simulink model "linear_model_with_controller"  (R2022b)
settings: Solver=VariableStepAuto  StartTime=0.0  StopTime=80  RelTol=1e-3
values from neighbouring files (symbols this model uses):
  A = [-3.78172659857e-08 0 0 0 2.97308e-08 0 0 0 0 1 5.79554624069e-35 6.21514719717e-19 ... (144 elements, 12x12)]    [A1.mat]    (also in A2.mat = [-3.78172659857e-08 0 0 0 2.97308e-08 0 0 0 0 1 -4.775625166; A3.mat = [-3.78172659857e-08 0 0 0 2.97308e-08 0 0 0 0 1 1.7488204834; A4.mat = [-3.78172659857e-08 0 0 0 2.97308e-08 0 0 0 0 1 -4.775625166)
  B = [-5.75123705385 0 0 0 10.0487888864 0 0 0 0 0 0 0 ... (48 elements, 12x4)]    [B1.mat]    (also in B2.mat = [-5.75123707143 0 0 0 10.0487889171 0 0 0 0 0 0 0 ... (48 el; B3.mat = [-5.75123705387 0 0 0 10.0487888865 0 0 0 0 0 0 0 ... (48 el; B4.mat = [-5.75123707143 0 0 0 10.0487889171 0 0 0 0 0 0 0 ... (48 el)
  Lcont = -inv(Sreg*Breg)*((Sreg*Areg)-(Phi*Sreg))*Tr    [Sliding_surface_design.m]
  S = [Mc eye(mm)]*Tr    [Sliding_surface_design.m]
undefined symbols (not defined in the file or in its folder): C, D
settings Model: Creator=henrr  LastModifiedBy=henrr
settings DataIOCC: SaveOutput=off  SaveTime=off  ReturnWorkspaceOutputs=off

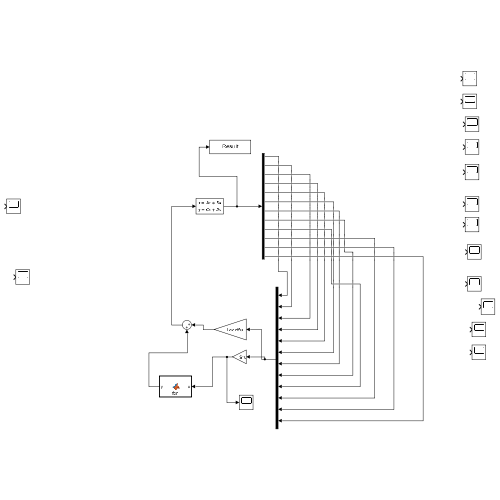
[thumbnail: Simulink's stored preview of the top-level diagram]
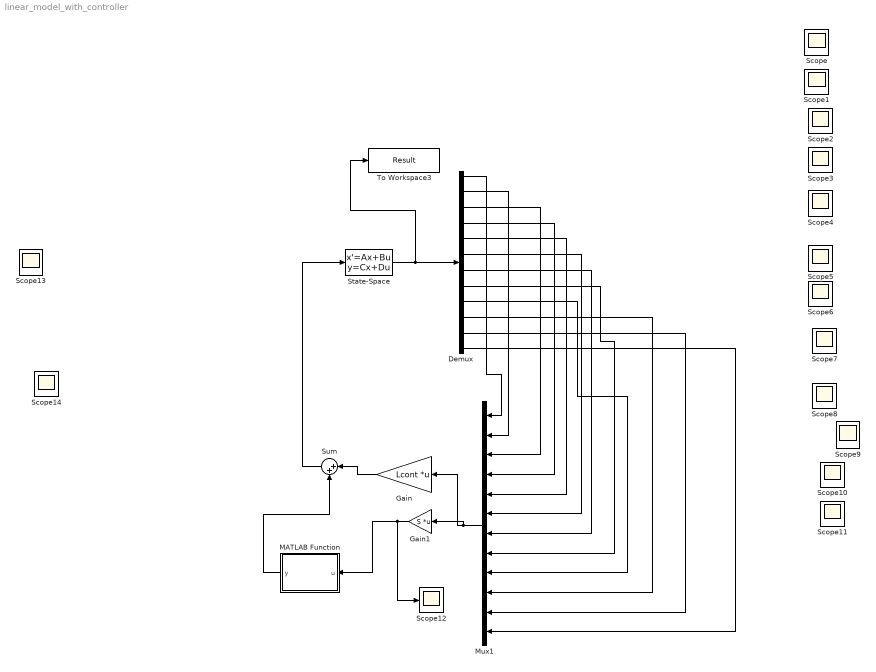
== system linear_model_with_controller ==
  Demux : Demux  Outputs=12
  Gain : Gain  Gain=Lcont  Multiplication=Matrix(K*u)
  Gain1 : Gain  Gain=S  Multiplication=Matrix(K*u)
  MATLAB Function : MATLAB Function  TreatAsAtomicUnit=on
  Mux1 : Mux  Inputs=12
  Scope{,1..14} (15 alike) : Scope
  State-Space : StateSpace  A=A  B=B  C=C  D=D  InitialCondition=[0.1,0,0,0,0,0,0,0,0,0,0,0]'  AllowTunableDMatrix=on
  Sum : Sum  Inputs=|++
  To Workspace3 : ToWorkspace  VariableName=Result  SaveFormat=Timeseries  SampleTime=-1
  wires:
  Demux/9 -> Mux1/9
  Demux/7 -> Mux1/7
  Demux/12 -> Mux1/12
  Demux/8 -> Mux1/8
  Demux/1 -> Mux1/1
  Demux/6 -> Mux1/6
  Demux/2 -> Mux1/2
  Demux/11 -> Mux1/11
  Demux/4 -> Mux1/4
  Demux/10 -> Mux1/10
  Demux/5 -> Mux1/5
  State-Space/1 -> To Workspace3/1, Demux/1
  Gain1/1 -> Scope12/1, MATLAB Function/1(u)
  Sum/1 -> State-Space/1
  Demux/3 -> Mux1/3
  Mux1/1 -> Gain1/1, Gain/1
  Gain/1 -> Sum/1
  MATLAB Function/1(y) -> Sum/2

== matlab function linear_model_with_controller/MATLAB Function ==
  data: u input; y output
function y = fcn(u)

 Lam=[11.5782    0.0000   -0.0000   -0.0000;
   -0.0000  -12.2181    0.0000   -0.0000;
    0.0000   -0.0000    0.6730    0.6449;
    0.0000   -0.0000   -0.0000   -0.4301];

P = [0.0250         0         0         0;
         0    0.0250         0         0;
         0         0    0.0250         0;
         0         0         0    0.0250;];

y = -10*inv(Lam)*P*u/(norm(P*u)+0.001);
